simulink model "case5"  (R2024b)
settings: Solver=FixedStepAuto  StartTime=0  StopTime=1  FixedStep=1e-7  RelTol=1e-3
values from neighbouring files (symbols this model uses):
  SG_D_1_D = 0.01056    [IEEE9_case_parameters.m]    (also in case1_parameters.m; case2_parameters.m; case3_parameters.m; case4_parameters.m)
  SG_D_1_EnableSaturation = 0    [IEEE9_case_parameters.m]    (also in case1_parameters.m; case2_parameters.m; case3_parameters.m; case4_parameters.m)
  SG_D_1_f0 = 60    [IEEE9_case_parameters.m]    (also in case1_parameters.m; case2_parameters.m; case3_parameters.m; case4_parameters.m)
  SG_D_1_H = 7.5    [IEEE9_case_parameters.m]    (also in case1_parameters.m; case2_parameters.m; case3_parameters.m; case4_parameters.m)
  SG_D_1_K_A = 20    [IEEE9_case_parameters.m]    (also in case1_parameters.m; case2_parameters.m; case3_parameters.m; case4_parameters.m)
  SG_D_1_K_E = 1.000000e+1    (= 10)    [IEEE9_case_parameters.m]    (also in case1_parameters.m; case2_parameters.m; case3_parameters.m; case4_parameters.m)
  SG_D_1_K_F = 2.363    [IEEE9_case_parameters.m]    (also in case1_parameters.m; case2_parameters.m; case3_parameters.m; case4_parameters.m)
  SG_D_1_K_s = 0.5    [IEEE9_case_parameters.m]    (also in case1_parameters.m = 5; case2_parameters.m = 5; case3_parameters.m = 5; case4_parameters.m = 5)
  SG_D_1_R_a = 0.001088    [IEEE9_case_parameters.m]    (also in case1_parameters.m; case2_parameters.m; case3_parameters.m; case4_parameters.m)
  SG_D_1_S_A = 1    [IEEE9_case_parameters.m]    (also in case1_parameters.m; case2_parameters.m; case3_parameters.m; case4_parameters.m)
  SG_D_1_S_B = 0.103    [IEEE9_case_parameters.m]    (also in case1_parameters.m; case2_parameters.m; case3_parameters.m; case4_parameters.m)
  SG_D_1_S_N = 10.659857    [IEEE9_case_parameters.m]    (also in case1_parameters.m; case2_parameters.m; case3_parameters.m; case4_parameters.m)
  SG_D_1_SpeedPara = 200    [IEEE9_case_parameters.m]    (also in case1_parameters.m; case2_parameters.m; case3_parameters.m; case4_parameters.m)
  SG_D_1_T_0 = 0.720173    [IEEE9_case_parameters.m]    (also in case1_parameters.m = 0.755522; case2_parameters.m = 0.808931; case3_parameters.m = 0.869402; case4_parameters.m = 0.729316)
  SG_D_1_T_1 = 0.3    [IEEE9_case_parameters.m]    (also in case1_parameters.m; case2_parameters.m; case3_parameters.m; case4_parameters.m)
  SG_D_1_T_2 = 0.05    [IEEE9_case_parameters.m]    (also in case1_parameters.m; case2_parameters.m; case3_parameters.m; case4_parameters.m)
  SG_D_1_T_3 = 0.02    [IEEE9_case_parameters.m]    (also in case1_parameters.m; case2_parameters.m; case3_parameters.m; case4_parameters.m)
  SG_D_1_T_4 = 0.005    [IEEE9_case_parameters.m]    (also in case1_parameters.m; case2_parameters.m; case3_parameters.m; case4_parameters.m)
  SG_D_1_T_A = 0.02    [IEEE9_case_parameters.m]    (also in case1_parameters.m; case2_parameters.m; case3_parameters.m; case4_parameters.m)
  SG_D_1_T_dd = 8.000000e+0    (= 8)    [IEEE9_case_parameters.m]    (also in case1_parameters.m; case2_parameters.m; case3_parameters.m; case4_parameters.m)
  SG_D_1_T_ddd = 0.04    [IEEE9_case_parameters.m]    (also in case1_parameters.m; case2_parameters.m; case3_parameters.m; case4_parameters.m)
  SG_D_1_T_E = 0.314    [IEEE9_case_parameters.m]    (also in case1_parameters.m; case2_parameters.m; case3_parameters.m; case4_parameters.m)
  SG_D_1_T_F = 0.35    [IEEE9_case_parameters.m]    (also in case1_parameters.m; case2_parameters.m; case3_parameters.m; case4_parameters.m)
  SG_D_1_T_qd = 0.8    [IEEE9_case_parameters.m]    (also in case1_parameters.m; case2_parameters.m; case3_parameters.m; case4_parameters.m)
  SG_D_1_T_qdd = 0.02    [IEEE9_case_parameters.m]    (also in case1_parameters.m; case2_parameters.m; case3_parameters.m; case4_parameters.m)
  SG_D_1_T_speed = 0.1    [IEEE9_case_parameters.m]    (also in case1_parameters.m = 200; case2_parameters.m = 200; case3_parameters.m = 200; case4_parameters.m = 200)
  SG_D_1_T_w = 0.5    [IEEE9_case_parameters.m]    (also in case1_parameters.m; case2_parameters.m; case3_parameters.m; case4_parameters.m)
  SG_D_1_V_ref = 1.990276    [IEEE9_case_parameters.m]    (also in case1_parameters.m = 2.042296; case2_parameters.m = 2.051388; case3_parameters.m = 2.089584; case4_parameters.m = 2.01845)
  SG_D_1_w_ref = 376.991118    [IEEE9_case_parameters.m]    (also in case1_parameters.m; case2_parameters.m; case3_parameters.m; case4_parameters.m)
  SG_D_1_wb = 6.000000e+1    (= 60)    [IEEE9_case_parameters.m]    (also in case1_parameters.m; case2_parameters.m; case3_parameters.m; case4_parameters.m)
  SG_D_1_x_d = 1.9    [IEEE9_case_parameters.m]    (also in case1_parameters.m; case2_parameters.m; case3_parameters.m; case4_parameters.m)
  SG_D_1_x_dd = 0.302    [IEEE9_case_parameters.m]    (also in case1_parameters.m; case2_parameters.m; case3_parameters.m; case4_parameters.m)
  SG_D_1_x_ddd = 0.204    [IEEE9_case_parameters.m]    (also in case1_parameters.m; case2_parameters.m; case3_parameters.m; case4_parameters.m)
  SG_D_1_x_l = 0.05    [IEEE9_case_parameters.m]    (also in case1_parameters.m; case2_parameters.m; case3_parameters.m; case4_parameters.m)
  SG_D_1_x_q = 1.3    [IEEE9_case_parameters.m]    (also in case1_parameters.m; case2_parameters.m; case3_parameters.m; case4_parameters.m)
  SG_D_1_x_qd = 0.5    [IEEE9_case_parameters.m]    (also in case1_parameters.m; case2_parameters.m; case3_parameters.m; case4_parameters.m)
  SG_D_1_x_qdd = 0.3    [IEEE9_case_parameters.m]    (also in case1_parameters.m; case2_parameters.m; case3_parameters.m; case4_parameters.m)
  SG_D_2_D = 0.02    [IEEE9_case_parameters.m]    (also in case1_parameters.m; case2_parameters.m; case3_parameters.m; case4_parameters.m)
  SG_D_2_EnableSaturation = 0    [IEEE9_case_parameters.m]    (also in case1_parameters.m; case2_parameters.m; case3_parameters.m; case4_parameters.m)
  SG_D_2_f0 = 60    [IEEE9_case_parameters.m]    (also in case1_parameters.m; case2_parameters.m; case3_parameters.m; case4_parameters.m)
  SG_D_2_H = 8.000000e+0    (= 8)    [IEEE9_case_parameters.m]    (also in case1_parameters.m; case2_parameters.m; case3_parameters.m; case4_parameters.m)
  SG_D_2_K_A = 20    [IEEE9_case_parameters.m]    (also in case1_parameters.m; case2_parameters.m; case3_parameters.m; case4_parameters.m)
  SG_D_2_K_E = 1.000000e+1    (= 10)    [IEEE9_case_parameters.m]    (also in case1_parameters.m; case2_parameters.m; case3_parameters.m; case4_parameters.m)
  SG_D_2_K_F = 2.363    [IEEE9_case_parameters.m]    (also in case1_parameters.m; case2_parameters.m; case3_parameters.m; case4_parameters.m)
  SG_D_2_K_s = 0.5    [IEEE9_case_parameters.m]    (also in case1_parameters.m = 4; case2_parameters.m = 4; case3_parameters.m = 4; case4_parameters.m = 4)
  SG_D_2_R_a = 0.001088    [IEEE9_case_parameters.m]    (also in case1_parameters.m; case2_parameters.m; case3_parameters.m; case4_parameters.m)
  SG_D_2_S_A = 1    [IEEE9_case_parameters.m]    (also in case1_parameters.m; case2_parameters.m; case3_parameters.m; case4_parameters.m)
  SG_D_2_S_B = 0.103    [IEEE9_case_parameters.m]    (also in case1_parameters.m; case2_parameters.m; case3_parameters.m; case4_parameters.m)
  SG_D_2_S_N = 10.659857    [IEEE9_case_parameters.m]    (also in case1_parameters.m; case2_parameters.m; case3_parameters.m; case4_parameters.m)
  SG_D_2_SpeedPara = 200    [IEEE9_case_parameters.m]    (also in case1_parameters.m; case2_parameters.m; case3_parameters.m; case4_parameters.m)
  SG_D_2_T_0 = 1.632913    [IEEE9_case_parameters.m]    (also in case1_parameters.m = 1.632925; case2_parameters.m = 1.632915; case3_parameters.m = 1.632914; case4_parameters.m = 1.632927)
  SG_D_2_T_1 = 0.2    [IEEE9_case_parameters.m]    (also in case1_parameters.m; case2_parameters.m; case3_parameters.m; case4_parameters.m)
  SG_D_2_T_2 = 0.05    [IEEE9_case_parameters.m]    (also in case1_parameters.m; case2_parameters.m; case3_parameters.m; case4_parameters.m)
  SG_D_2_T_3 = 0.02    [IEEE9_case_parameters.m]    (also in case1_parameters.m; case2_parameters.m; case3_parameters.m; case4_parameters.m)
  SG_D_2_T_4 = 0.005    [IEEE9_case_parameters.m]    (also in case1_parameters.m; case2_parameters.m; case3_parameters.m; case4_parameters.m)
  SG_D_2_T_A = 0.02    [IEEE9_case_parameters.m]    (also in case1_parameters.m; case2_parameters.m; case3_parameters.m; case4_parameters.m)
  SG_D_2_T_dd = 7.9    [IEEE9_case_parameters.m]    (also in case1_parameters.m; case2_parameters.m; case3_parameters.m; case4_parameters.m)
  SG_D_2_T_ddd = 0.04    [IEEE9_case_parameters.m]    (also in case1_parameters.m; case2_parameters.m; case3_parameters.m; case4_parameters.m)
  SG_D_2_T_E = 0.314    [IEEE9_case_parameters.m]    (also in case1_parameters.m; case2_parameters.m; case3_parameters.m; case4_parameters.m)
  SG_D_2_T_F = 0.35    [IEEE9_case_parameters.m]    (also in case1_parameters.m; case2_parameters.m; case3_parameters.m; case4_parameters.m)
  SG_D_2_T_qd = 0.8    [IEEE9_case_parameters.m]    (also in case1_parameters.m; case2_parameters.m; case3_parameters.m; case4_parameters.m)
  SG_D_2_T_qdd = 0.015    [IEEE9_case_parameters.m]    (also in case1_parameters.m; case2_parameters.m; case3_parameters.m; case4_parameters.m)
  SG_D_2_T_speed = 0.1    [IEEE9_case_parameters.m]    (also in case1_parameters.m = 150; case2_parameters.m = 150; case3_parameters.m = 150; case4_parameters.m = 150)
  SG_D_2_T_w = 0.35    [IEEE9_case_parameters.m]    (also in case1_parameters.m; case2_parameters.m; case3_parameters.m; case4_parameters.m)
  SG_D_2_V_ref = 2.58547    [IEEE9_case_parameters.m]    (also in case1_parameters.m = 2.597896; case2_parameters.m = 2.587136; case3_parameters.m = 2.586042; case4_parameters.m = 2.599679)
  SG_D_2_w_ref = 376.991118    [IEEE9_case_parameters.m]    (also in case1_parameters.m; case2_parameters.m; case3_parameters.m; case4_parameters.m)
  SG_D_2_wb = 6.000000e+1    (= 60)    [IEEE9_case_parameters.m]    (also in case1_parameters.m; case2_parameters.m; case3_parameters.m; case4_parameters.m)
  SG_D_2_x_d = 1.8    [IEEE9_case_parameters.m]    (also in case1_parameters.m; case2_parameters.m; case3_parameters.m; case4_parameters.m)
  SG_D_2_x_dd = 0.302    [IEEE9_case_parameters.m]    (also in case1_parameters.m; case2_parameters.m; case3_parameters.m; case4_parameters.m)
  SG_D_2_x_ddd = 0.204    [IEEE9_case_parameters.m]    (also in case1_parameters.m; case2_parameters.m; case3_parameters.m; case4_parameters.m)
  SG_D_2_x_l = 0.05    [IEEE9_case_parameters.m]    (also in case1_parameters.m; case2_parameters.m; case3_parameters.m; case4_parameters.m)
  SG_D_2_x_q = 1.25    [IEEE9_case_parameters.m]    (also in case1_parameters.m; case2_parameters.m; case3_parameters.m; case4_parameters.m)
  SG_D_2_x_qd = 0.5    [IEEE9_case_parameters.m]    (also in case1_parameters.m; case2_parameters.m; case3_parameters.m; case4_parameters.m)
  SG_D_2_x_qdd = 0.3    [IEEE9_case_parameters.m]    (also in case1_parameters.m; case2_parameters.m; case3_parameters.m; case4_parameters.m)
  SG_D_3_D = 0.02    [IEEE9_case_parameters.m]    (also in case1_parameters.m; case2_parameters.m; case3_parameters.m; case4_parameters.m)
  SG_D_3_EnableSaturation = 0    [IEEE9_case_parameters.m]    (also in case1_parameters.m; case2_parameters.m; case3_parameters.m; case4_parameters.m)
  SG_D_3_f0 = 60    [IEEE9_case_parameters.m]    (also in case1_parameters.m; case2_parameters.m; case3_parameters.m; case4_parameters.m)
  SG_D_3_H = 7.7    [IEEE9_case_parameters.m]    (also in case1_parameters.m; case2_parameters.m; case3_parameters.m; case4_parameters.m)
  SG_D_3_K_A = 20    [IEEE9_case_parameters.m]    (also in case1_parameters.m; case2_parameters.m; case3_parameters.m; case4_parameters.m)
  SG_D_3_K_E = 1.000000e+1    (= 10)    [IEEE9_case_parameters.m]    (also in case1_parameters.m; case2_parameters.m; case3_parameters.m; case4_parameters.m)
  SG_D_3_K_F = 2.363    [IEEE9_case_parameters.m]    (also in case1_parameters.m; case2_parameters.m; case3_parameters.m; case4_parameters.m)
  SG_D_3_K_s = 0.2    [IEEE9_case_parameters.m]    (also in case1_parameters.m = 2; case2_parameters.m = 2; case3_parameters.m = 2; case4_parameters.m = 2)
  SG_D_3_R_a = 0.001088    [IEEE9_case_parameters.m]    (also in case1_parameters.m; case2_parameters.m; case3_parameters.m; case4_parameters.m)
  SG_D_3_S_A = 1    [IEEE9_case_parameters.m]    (also in case1_parameters.m; case2_parameters.m; case3_parameters.m; case4_parameters.m)
  SG_D_3_S_B = 0.103    [IEEE9_case_parameters.m]    (also in case1_parameters.m; case2_parameters.m; case3_parameters.m; case4_parameters.m)
  SG_D_3_S_N = 10.659857    [IEEE9_case_parameters.m]    (also in case1_parameters.m; case2_parameters.m; case3_parameters.m; case4_parameters.m)
  SG_D_3_SpeedPara = 200    [IEEE9_case_parameters.m]    (also in case1_parameters.m; case2_parameters.m; case3_parameters.m; case4_parameters.m)
  SG_D_3_T_0 = 0.850788    [IEEE9_case_parameters.m]    (also in case1_parameters.m = 0.850786; case2_parameters.m = 0.850787; case3_parameters.m; case4_parameters.m = 0.850786)
  SG_D_3_T_1 = 0.2    [IEEE9_case_parameters.m]    (also in case1_parameters.m; case2_parameters.m; case3_parameters.m; case4_parameters.m)
  SG_D_3_T_2 = 0.05    [IEEE9_case_parameters.m]    (also in case1_parameters.m; case2_parameters.m; case3_parameters.m; case4_parameters.m)
  SG_D_3_T_3 = 0.02    [IEEE9_case_parameters.m]    (also in case1_parameters.m; case2_parameters.m; case3_parameters.m; case4_parameters.m)
  SG_D_3_T_4 = 0.005    [IEEE9_case_parameters.m]    (also in case1_parameters.m; case2_parameters.m; case3_parameters.m; case4_parameters.m)
  SG_D_3_T_A = 0.02    [IEEE9_case_parameters.m]    (also in case1_parameters.m; case2_parameters.m; case3_parameters.m; case4_parameters.m)
  SG_D_3_T_dd = 8.1    [IEEE9_case_parameters.m]    (also in case1_parameters.m; case2_parameters.m; case3_parameters.m; case4_parameters.m)
  SG_D_3_T_ddd = 0.04    [IEEE9_case_parameters.m]    (also in case1_parameters.m; case2_parameters.m; case3_parameters.m; case4_parameters.m)
  SG_D_3_T_E = 0.314    [IEEE9_case_parameters.m]    (also in case1_parameters.m; case2_parameters.m; case3_parameters.m; case4_parameters.m)
  SG_D_3_T_F = 0.35    [IEEE9_case_parameters.m]    (also in case1_parameters.m; case2_parameters.m; case3_parameters.m; case4_parameters.m)
  SG_D_3_T_qd = 0.8    [IEEE9_case_parameters.m]    (also in case1_parameters.m; case2_parameters.m; case3_parameters.m; case4_parameters.m)
  SG_D_3_T_qdd = 0.015    [IEEE9_case_parameters.m]    (also in case1_parameters.m; case2_parameters.m; case3_parameters.m; case4_parameters.m)
  SG_D_3_T_speed = 0.1    [IEEE9_case_parameters.m]    (also in case1_parameters.m = 180; case2_parameters.m = 180; case3_parameters.m = 180; case4_parameters.m = 180)
  SG_D_3_T_w = 0.4    [IEEE9_case_parameters.m]    (also in case1_parameters.m; case2_parameters.m; case3_parameters.m; case4_parameters.m)
  SG_D_3_V_ref = 1.892727    [IEEE9_case_parameters.m]    (also in case1_parameters.m = 1.906439; case2_parameters.m = 1.895535; case3_parameters.m = 1.892105; case4_parameters.m = 1.906598)
  SG_D_3_w_ref = 376.991118    [IEEE9_case_parameters.m]    (also in case1_parameters.m; case2_parameters.m; case3_parameters.m; case4_parameters.m)
  SG_D_3_wb = 6.000000e+1    (= 60)    [IEEE9_case_parameters.m]    (also in case1_parameters.m; case2_parameters.m; case3_parameters.m; case4_parameters.m)
  SG_D_3_x_d = 1.85    [IEEE9_case_parameters.m]    (also in case1_parameters.m; case2_parameters.m; case3_parameters.m; case4_parameters.m)
  SG_D_3_x_dd = 0.302    [IEEE9_case_parameters.m]    (also in case1_parameters.m; case2_parameters.m; case3_parameters.m; case4_parameters.m)
  SG_D_3_x_ddd = 0.204    [IEEE9_case_parameters.m]    (also in case1_parameters.m; case2_parameters.m; case3_parameters.m; case4_parameters.m)
  SG_D_3_x_l = 0.05    [IEEE9_case_parameters.m]    (also in case1_parameters.m; case2_parameters.m; case3_parameters.m; case4_parameters.m)
  SG_D_3_x_q = 1.2    [IEEE9_case_parameters.m]    (also in case1_parameters.m; case2_parameters.m; case3_parameters.m; case4_parameters.m)
  SG_D_3_x_qd = 0.5    [IEEE9_case_parameters.m]    (also in case1_parameters.m; case2_parameters.m; case3_parameters.m; case4_parameters.m)
  SG_D_3_x_qdd = 0.3    [IEEE9_case_parameters.m]    (also in case1_parameters.m; case2_parameters.m; case3_parameters.m; case4_parameters.m)
(part 7 of 12)

== system case5/SG_D_2/T_e_SG_D_2_block ==
  note: T_e_SG_D_2 in case5
      | $-\frac{\psi _{d,\mathrm{SG},D,2}\,\left(\psi _{q,\mathrm{SG},D,2}+\frac{\psi _{\mathrm{gq},\mathrm{SG},D,2}\,\left(x_{l}-x_{\mathrm{qdd}}\right)}{x_{l}-x_{\mathrm{qd}}}+\frac{\psi _{\mathrm{kq},\mathrm{SG},D,2}\,\left(x_{\mathrm{qd}}-x_{\mathrm{qdd}}\right)}{x_{l}-x_{\mathrm{qd}}}\right)}{x_{\mathrm{qdd}}}-\frac{\psi _{q,\mathrm{SG},D,2}\,\left(\frac{\psi _{\mathrm{1d},\mathrm{SG},D,2}\,\left(x_{\mathrm{dd}}-x_{\mathrm{ddd}}\right)}{x_{\mathrm{dd}}-x_{l}}-\psi _{d,\mathrm{SG},D,2}+\frac{\psi _{\mathrm{fd},\mathrm{SG},D,2}\,\left(x_{\mathrm{ddd}}-x_{l}\right)}{x_{\mathrm{dd}}-x_{l}}\right)}{x_{\mathrm{ddd}}}$
      | Automatically generated on 2025-10-31 19:11:59 .
  State_psi_d_SG_D_2_8764f : Inport
  State_psi_gq_SG_D_2_1f7cf : Inport  Port=2
  State_psi_kq_SG_D_2_b1f64 : Inport  Port=3
  State_psi_q_SG_D_2_7d7d0 : Inport  Port=4
  State_psi_q_SG_D_2_860cc : Inport  Port=5
  State_psi_1d_SG_D_2_4989b : Inport  Port=6
  State_psi_d_SG_D_2_cc96c : Inport  Port=7
  State_psi_fd_SG_D_2_f288a : Inport  Port=8
  Add_4ea1b : Sum
  Add_6a2e1 : Sum
  Add_77a1d : Sum
  Add_7defb : Sum
  Add_a1766 : Sum
  Add_fd560 : Sum
  Constant_-1_6d645 : Constant  Value=-1
  Constant_-1_6fd96 : Constant  Value=-1
  Constant_-1_a2653 : Constant  Value=-1
  Constant_-1_bed53 : Constant  Value=-1
  Constant_-1_c9aec : Constant  Value=-1
  Constant_x_dd_110ca : Constant  Value=x_dd
  Constant_x_dd_1b426 : Constant  Value=x_dd
  Constant_x_dd_603c3 : Constant  Value=x_dd
  Constant_x_ddd_039fd : Constant  Value=x_ddd
  Constant_x_ddd_2ebf2 : Constant  Value=x_ddd
  Constant_x_ddd_fde4e : Constant  Value=x_ddd
  Constant_x_l_026ea : Constant  Value=x_l
  Constant_x_l_085f5 : Constant  Value=x_l
  Constant_x_l_13a0c : Constant  Value=x_l
  Constant_x_l_3979a : Constant  Value=x_l
  Constant_x_l_ba3c7 : Constant  Value=x_l
  Constant_x_l_ec106 : Constant  Value=x_l
  Constant_x_qd_460b0 : Constant  Value=x_qd
  Constant_x_qd_54b57 : Constant  Value=x_qd
  Constant_x_qd_ab5a4 : Constant  Value=x_qd
  Constant_x_qdd_30d29 : Constant  Value=x_qdd
  Constant_x_qdd_b0a37 : Constant  Value=x_qdd
  Constant_x_qdd_b570c : Constant  Value=x_qdd
  Divide_13c40 : Product  Inputs=*/
  Divide_4a1e5 : Product  Inputs=*/
  Divide_838a3 : Product  Inputs=*/
  Divide_9315b : Product  Inputs=*/
  Divide_db35b : Product  Inputs=*/
  Divide_fdf5d : Product  Inputs=*/
  Product_176e1 : Product
  Product_33191 : Product
  Product_43418 : Product
  Product_7e007 : Product
  Product_84689 : Product
  Product_85a87 : Product
  Product_8d2ff : Product
  Product_a5a2e : Product
  Product_ac49e : Product
  Product_b4402 : Product
  Product_dabe4 : Product
  Subtract_0e07a : Sum  Inputs=+-
  Subtract_45d12 : Sum  Inputs=+-
  Subtract_70a71 : Sum  Inputs=+-
  Subtract_7eb8f : Sum  Inputs=+-
  Subtract_970c6 : Sum  Inputs=+-
  Subtract_e5e99 : Sum  Inputs=+-
  Subtract_ef4a2 : Sum  Inputs=+-
  Blockout_T_e_SG_D_2_32ea4 : Outport
  wires:
  Constant_-1_6fd96/1 -> Product_7e007/1
  Divide_fdf5d/1 -> Subtract_e5e99/1
  Constant_-1_bed53/1 -> Product_176e1/1
  Constant_x_l_085f5/1 -> Product_176e1/2
  Constant_x_qd_460b0/1 -> Subtract_45d12/1
  Product_33191/1 -> Divide_fdf5d/1
  Product_176e1/1 -> Add_6a2e1/1
  Divide_13c40/1 -> Subtract_970c6/2
  Constant_x_qdd_b0a37/1 -> Subtract_45d12/2
  Constant_x_qdd_30d29/1 -> Divide_4a1e5/2
  Constant_x_ddd_2ebf2/1 -> Subtract_7eb8f/2
  Constant_x_qdd_b570c/1 -> Add_6a2e1/2
  Constant_x_l_ba3c7/1 -> Product_7e007/2
  Constant_-1_c9aec/1 -> Product_84689/1
  Constant_x_l_3979a/1 -> Product_84689/2
  Constant_-1_a2653/1 -> Product_8d2ff/1
  State_psi_1d_SG_D_2_4989b/1 -> Product_8d2ff/2
  Constant_x_dd_603c3/1 -> Subtract_7eb8f/1
  Divide_db35b/1 -> Subtract_e5e99/2
  State_psi_gq_SG_D_2_1f7cf/1 -> Product_33191/1
  Add_6a2e1/1 -> Product_33191/2
  Subtract_e5e99/1 -> Add_a1766/1
  Constant_x_dd_1b426/1 -> Subtract_ef4a2/1
  Product_7e007/1 -> Add_4ea1b/1
  Product_43418/1 -> Product_b4402/1
  Constant_x_qd_ab5a4/1 -> Add_4ea1b/2
  State_psi_kq_SG_D_2_b1f64/1 -> Product_dabe4/1
  Subtract_45d12/1 -> Product_dabe4/2
  Product_84689/1 -> Add_77a1d/1
  State_psi_q_SG_D_2_860cc/1 -> Product_ac49e/1
  Constant_x_qd_54b57/1 -> Add_77a1d/2
  Product_8d2ff/1 -> Product_85a87/1
  Divide_9315b/1 -> Add_7defb/2
  Subtract_7eb8f/1 -> Product_85a87/2
  Constant_x_l_13a0c/1 -> Subtract_ef4a2/2
  Constant_x_ddd_039fd/1 -> Subtract_70a71/1
  Constant_x_dd_110ca/1 -> Subtract_0e07a/1
  Constant_x_l_ec106/1 -> Subtract_70a71/2
  Add_7defb/1 -> Blockout_T_e_SG_D_2_32ea4/1
  Add_4ea1b/1 -> Divide_fdf5d/2
  Product_dabe4/1 -> Divide_db35b/1
  Product_b4402/1 -> Divide_4a1e5/1
  State_psi_d_SG_D_2_8764f/1 -> Product_43418/2
  Add_77a1d/1 -> Divide_db35b/2
  Product_85a87/1 -> Divide_838a3/1
  Subtract_ef4a2/1 -> Divide_838a3/2
  Constant_x_l_026ea/1 -> Subtract_0e07a/2
  State_psi_fd_SG_D_2_f288a/1 -> Product_a5a2e/1
  Constant_x_ddd_fde4e/1 -> Divide_9315b/2
  Product_ac49e/1 -> Divide_9315b/1
  Subtract_70a71/1 -> Product_a5a2e/2
  Divide_838a3/1 -> Add_fd560/1
  State_psi_d_SG_D_2_cc96c/1 -> Add_fd560/2
  Add_fd560/1 -> Subtract_970c6/1
  Product_a5a2e/1 -> Divide_13c40/1
  Subtract_0e07a/1 -> Divide_13c40/2
  Constant_-1_6d645/1 -> Product_43418/1
  State_psi_q_SG_D_2_7d7d0/1 -> Add_a1766/2
  Add_a1766/1 -> Product_b4402/2
  Subtract_970c6/1 -> Product_ac49e/2
  Divide_4a1e5/1 -> Add_7defb/1

== system case5/SG_D_2/d_E_fd_SG_D_2_block ==
  note: d_E_fd_SG_D_2 in case5
      | $\frac{V_{f,\mathrm{SG},D,2}-E_{\mathrm{fd},\mathrm{SG},D,2}\,K_{E}}{T_{E}}$
      | Automatically generated on 2025-10-31 19:11:39 .
  State_E_fd_SG_D_2_808fd : Inport
  State_V_f_SG_D_2_4e077 : Inport  Port=2
  Add_b92ab : Sum
  Constant_-1_6f407 : Constant  Value=-1
  Constant_K_E_a9583 : Constant  Value=K_E
  Constant_T_E_299c6 : Constant  Value=T_E
  Divide_a8a3d : Product  Inputs=*/
  Product_10ad6 : Product
  Product_f58d4 : Product
  Blockout_d_E_fd_SG_D_2_55c73 : Outport
  wires:
  Constant_-1_6f407/1 -> Product_f58d4/1
  State_E_fd_SG_D_2_808fd/1 -> Product_f58d4/2
  Product_f58d4/1 -> Product_10ad6/1
  Constant_K_E_a9583/1 -> Product_10ad6/2
  Product_10ad6/1 -> Add_b92ab/1
  Constant_T_E_299c6/1 -> Divide_a8a3d/2
  State_V_f_SG_D_2_4e077/1 -> Add_b92ab/2
  Add_b92ab/1 -> Divide_a8a3d/1
  Divide_a8a3d/1 -> Blockout_d_E_fd_SG_D_2_55c73/1

== system case5/SG_D_2/d_Px_1_SG_D_2_block ==
  note: d_Px_1_SG_D_2 in case5
      | $\frac{w_{\mathrm{SG},D,2}-2\,\pi \,f_{0}}{T_{w}}-\frac{\mathrm{Px}_{1,\mathrm{SG},D,2}}{T_{w}}$
      | Automatically generated on 2025-10-31 19:11:41 .
  State_Px_1_SG_D_2_dcfec : Inport
  State_w_SG_D_2_0a872 : Inport  Port=2
  Add_7fc50 : Sum
  Add_fd0af : Sum
  Constant_-1_18e10 : Constant  Value=-1
  Constant_-2.0_af387 : Constant  Value=-2.0
  Constant_T_w_4ffa8 : Constant  Value=T_w
  Constant_T_w_f48b1 : Constant  Value=T_w
  Constant_f0_97983 : Constant  Value=f0
  Constant_pi_be5bb : Constant  Value=pi
  Divide_2a4bc : Product  Inputs=*/
  Divide_789a1 : Product  Inputs=*/
  Product_0c877 : Product
  Product_1a8c9 : Product
  Product_e895c : Product
  Blockout_d_Px_1_SG_D_2_3a836 : Outport
  wires:
  Constant_-2.0_af387/1 -> Product_1a8c9/1
  State_w_SG_D_2_0a872/1 -> Add_fd0af/2
  Constant_pi_be5bb/1 -> Product_1a8c9/2
  Product_1a8c9/1 -> Product_e895c/1
  Constant_f0_97983/1 -> Product_e895c/2
  Constant_-1_18e10/1 -> Product_0c877/1
  State_Px_1_SG_D_2_dcfec/1 -> Product_0c877/2
  Product_e895c/1 -> Add_fd0af/1
  Product_0c877/1 -> Divide_2a4bc/1
  Constant_T_w_4ffa8/1 -> Divide_2a4bc/2
  Add_fd0af/1 -> Divide_789a1/1
  Constant_T_w_f48b1/1 -> Divide_789a1/2
  Divide_2a4bc/1 -> Add_7fc50/1
  Divide_789a1/1 -> Add_7fc50/2
  Add_7fc50/1 -> Blockout_d_Px_1_SG_D_2_3a836/1

== system case5/SG_D_2/d_Px_2_SG_D_2_block ==
  note: d_Px_2_SG_D_2 in case5
      | $\frac{\mathrm{Px}_{1,\mathrm{SG},D,2}-T_{2}\,\left(\frac{\mathrm{Px}_{1,\mathrm{SG},D,2}}{T_{w}}-\frac{w_{\mathrm{SG},D,2}-2\,\pi \,f_{0}}{T_{w}}\right)}{T_{1}}-\frac{\mathrm{Px}_{2,\mathrm{SG},D,2}}{T_{1}}$
      | Automatically generated on 2025-10-31 19:11:43 .
  State_Px_2_SG_D_2_3d84e : Inport
  State_Px_1_SG_D_2_e7928 : Inport  Port=2
  State_Px_1_SG_D_2_6b838 : Inport  Port=3
  State_w_SG_D_2_c4bce : Inport  Port=4
  Add_00813 : Sum
  Add_8757f : Sum
  Add_8a97d : Sum
  Add_952a4 : Sum
  Constant_-1_2daee : Constant  Value=-1
  Constant_-1_d1ca8 : Constant  Value=-1
  Constant_-2.0_4ab62 : Constant  Value=-2.0
  Constant_T_1_280f9 : Constant  Value=T_1
  Constant_T_1_6f68d : Constant  Value=T_1
  Constant_T_2_6ecb6 : Constant  Value=T_2
  Constant_T_w_041db : Constant  Value=T_w
  Constant_T_w_4627f : Constant  Value=T_w
  Constant_f0_1ecde : Constant  Value=f0
  Constant_pi_53a50 : Constant  Value=pi
  Divide_01d62 : Product  Inputs=*/
  Divide_210ef : Product  Inputs=*/
  Divide_4f18f : Product  Inputs=*/
  Divide_ac4e2 : Product  Inputs=*/
  Product_3c12f : Product
  Product_6f61c : Product
  Product_9cbe4 : Product
  Product_a935b : Product
  Product_be960 : Product
  Blockout_d_Px_2_SG_D_2_04e36 : Outport
  wires:
  Constant_-1_d1ca8/1 -> Product_9cbe4/1
  Constant_-2.0_4ab62/1 -> Product_3c12f/1
  Product_be960/1 -> Add_952a4/2
  State_w_SG_D_2_c4bce/1 -> Add_8a97d/2
  Constant_pi_53a50/1 -> Product_3c12f/2
  Product_3c12f/1 -> Product_a935b/1
  State_Px_1_SG_D_2_6b838/1 -> Product_6f61c/2
  Constant_f0_1ecde/1 -> Product_a935b/2
  State_Px_2_SG_D_2_3d84e/1 -> Product_9cbe4/2
  Constant_-1_2daee/1 -> Product_6f61c/1
  Product_a935b/1 -> Add_8a97d/1
  Product_6f61c/1 -> Divide_210ef/1
  Constant_T_w_041db/1 -> Divide_210ef/2
  Add_8a97d/1 -> Divide_4f18f/1
  Constant_T_w_4627f/1 -> Divide_4f18f/2
  Divide_210ef/1 -> Add_8757f/1
  Divide_4f18f/1 -> Add_8757f/2
  Constant_T_2_6ecb6/1 -> Product_be960/1
  Add_8757f/1 -> Product_be960/2
  State_Px_1_SG_D_2_e7928/1 -> Add_952a4/1
  Product_9cbe4/1 -> Divide_ac4e2/1
  Constant_T_1_280f9/1 -> Divide_ac4e2/2
  Add_952a4/1 -> Divide_01d62/1
  Constant_T_1_6f68d/1 -> Divide_01d62/2
  Divide_ac4e2/1 -> Add_00813/1
  Divide_01d62/1 -> Add_00813/2
  Add_00813/1 -> Blockout_d_Px_2_SG_D_2_04e36/1

== system case5/SG_D_2/d_Px_3_SG_D_2_block ==
  note: d_Px_3_SG_D_2 in case5
      | $\frac{\mathrm{Px}_{2,\mathrm{SG},D,2}+T_{4}\,\left(\frac{\mathrm{Px}_{1,\mathrm{SG},D,2}-T_{2}\,\left(\frac{\mathrm{Px}_{1,\mathrm{SG},D,2}}{T_{w}}-\frac{w_{\mathrm{SG},D,2}-2\,\pi \,f_{0}}{T_{w}}\right)}{T_{1}}-\frac{\mathrm{Px}_{2,\mathrm{SG},D,2}}{T_{1}}\right)}{T_{3}}-\frac{\mathrm{Px}_{3,\mathrm{SG},D,2}}{T_{3}}$
      | Automatically generated on 2025-10-31 19:11:45 .
  State_Px_3_SG_D_2_615b8 : Inport
  State_Px_2_SG_D_2_ea741 : Inport  Port=2
  State_Px_2_SG_D_2_55edc : Inport  Port=3
  State_Px_1_SG_D_2_820be : Inport  Port=4
  State_Px_1_SG_D_2_81adf : Inport  Port=5
  State_w_SG_D_2_e9070 : Inport  Port=6
  Add_0c02d : Sum
  Add_3158f : Sum
  Add_4fdfa : Sum
  Add_6455c : Sum
  Add_eabaa : Sum
  Add_f9b5f : Sum
  Constant_-1_9126a : Constant  Value=-1
  Constant_-1_9489f : Constant  Value=-1
  Constant_-1_ca78e : Constant  Value=-1
  Constant_-2.0_ac31e : Constant  Value=-2.0
  Constant_T_1_10029 : Constant  Value=T_1
  Constant_T_1_13c66 : Constant  Value=T_1
  Constant_T_2_c8116 : Constant  Value=T_2
  Constant_T_3_c6817 : Constant  Value=T_3
  Constant_T_3_d860c : Constant  Value=T_3
  Constant_T_4_9c252 : Constant  Value=T_4
  Constant_T_w_8815c : Constant  Value=T_w
  Constant_T_w_ab9ec : Constant  Value=T_w
  Constant_f0_cbd55 : Constant  Value=f0
  Constant_pi_70a46 : Constant  Value=pi
  Divide_1514f : Product  Inputs=*/
  Divide_1df3f : Product  Inputs=*/
  Divide_2f4db : Product  Inputs=*/
  Divide_36895 : Product  Inputs=*/
  Divide_9d579 : Product  Inputs=*/
  Divide_addd2 : Product  Inputs=*/
  Product_8d7a1 : Product
  Product_b1d42 : Product
  Product_b6660 : Product
  Product_ba740 : Product
  Product_d1cf8 : Product
  Product_ee23a : Product
  Product_fb85f : Product
  Blockout_d_Px_3_SG_D_2_0e921 : Outport
  wires:
  Constant_-2.0_ac31e/1 -> Product_8d7a1/1
  State_w_SG_D_2_e9070/1 -> Add_4fdfa/2
  Add_eabaa/1 -> Divide_2f4db/1
  Constant_pi_70a46/1 -> Product_8d7a1/2
  Constant_-1_9489f/1 -> Product_fb85f/1
  Product_8d7a1/1 -> Product_b1d42/1
  State_Px_2_SG_D_2_55edc/1 -> Product_fb85f/2
  State_Px_1_SG_D_2_81adf/1 -> Product_d1cf8/2
  Divide_2f4db/1 -> Add_f9b5f/2
  Constant_f0_cbd55/1 -> Product_b1d42/2
  Constant_-1_9126a/1 -> Product_d1cf8/1
  Product_b1d42/1 -> Add_4fdfa/1
  Product_d1cf8/1 -> Divide_1df3f/1
  Constant_T_w_8815c/1 -> Divide_1df3f/2
  Divide_1514f/1 -> Add_f9b5f/1
  Add_4fdfa/1 -> Divide_36895/1
  Product_b6660/1 -> Add_0c02d/2
  Constant_T_w_ab9ec/1 -> Divide_36895/2
  Divide_1df3f/1 -> Add_6455c/1
  State_Px_1_SG_D_2_820be/1 -> Add_0c02d/1
  Divide_36895/1 -> Add_6455c/2
  Constant_-1_ca78e/1 -> Product_ee23a/1
  Constant_T_2_c8116/1 -> Product_b6660/1
  Add_6455c/1 -> Product_b6660/2
  Product_fb85f/1 -> Divide_9d579/1
  Constant_T_1_13c66/1 -> Divide_9d579/2
  Add_0c02d/1 -> Divide_addd2/1
  Constant_T_1_10029/1 -> Divide_addd2/2
  Divide_9d579/1 -> Add_3158f/1
  Divide_addd2/1 -> Add_3158f/2
  Constant_T_4_9c252/1 -> Product_ba740/1
  Add_3158f/1 -> Product_ba740/2
  State_Px_3_SG_D_2_615b8/1 -> Product_ee23a/2
  State_Px_2_SG_D_2_ea741/1 -> Add_eabaa/1
  Product_ba740/1 -> Add_eabaa/2
  Product_ee23a/1 -> Divide_1514f/1
  Constant_T_3_c6817/1 -> Divide_1514f/2
  Constant_T_3_d860c/1 -> Divide_2f4db/2
  Add_f9b5f/1 -> Blockout_d_Px_3_SG_D_2_0e921/1

== system case5/SG_D_2/d_R_f_SG_D_2_block ==
  note: d_R_f_SG_D_2 in case5
      | $-\frac{R_{f,\mathrm{SG},D,2}-\frac{E_{\mathrm{fd},\mathrm{SG},D,2}\,K_{F}}{T_{F}}}{T_{F}}$
      | Automatically generated on 2025-10-31 19:11:38 .
  State_E_fd_SG_D_2_65d60 : Inport
  State_R_f_SG_D_2_625bf : Inport  Port=2
  Constant_K_F_8c078 : Constant  Value=K_F
  Constant_T_F_a58c1 : Constant  Value=T_F
  Constant_T_F_f09bb : Constant  Value=T_F
  Divide_3b7b4 : Product  Inputs=*/
  Divide_81cba : Product  Inputs=*/
  Product_37f63 : Product
  Subtract_38e20 : Sum  Inputs=+-
  Blockout_d_R_f_SG_D_2_818dd : Outport
  wires:
  Constant_T_F_f09bb/1 -> Divide_3b7b4/2
  State_E_fd_SG_D_2_65d60/1 -> Product_37f63/1
  Constant_K_F_8c078/1 -> Product_37f63/2
  State_R_f_SG_D_2_625bf/1 -> Subtract_38e20/2
  Product_37f63/1 -> Divide_3b7b4/1
  Divide_3b7b4/1 -> Subtract_38e20/1
  Constant_T_F_a58c1/1 -> Divide_81cba/2
  Subtract_38e20/1 -> Divide_81cba/1
  Divide_81cba/1 -> Blockout_d_R_f_SG_D_2_818dd/1

== system case5/SG_D_2/d_T_m_SG_D_2_block ==
  note: d_T_m_SG_D_2 in case5
      | $-\frac{T_{m,\mathrm{SG},D,2}-T_{0}+\frac{\mathrm{SpeedPara}\,\left(w_{\mathrm{SG},D,2}-w_{\mathrm{ref}}\right)}{2\,f_{0}\,\pi }}{T_{\mathrm{speed}}}$
      | Automatically generated on 2025-10-31 19:11:28 .
  State_w_SG_D_2_ee856 : Inport
  State_T_m_SG_D_2_0b68a : Inport  Port=2
  Add_4c623 : Sum
  Add_d7e7d : Sum
  Constant_-1_7beba : Constant  Value=-1
  Constant_2.0_8024e : Constant  Value=2.0
  Constant_SpeedPara_13d3b : Constant  Value=SpeedPara
  Constant_T_0_5f1eb : Constant  Value=T_0
  Constant_T_speed_bed5c : Constant  Value=T_speed
  Constant_f0_62c1f : Constant  Value=f0
  Constant_pi_14469 : Constant  Value=pi
  Constant_w_ref_ef544 : Constant  Value=w_ref
  Divide_f0042 : Product  Inputs=*/
  Divide_f2c70 : Product  Inputs=*/
  Product_093fa : Product
  Product_6154c : Product
  Product_c4892 : Product
  Product_c5360 : Product
  Subtract_f335a : Sum  Inputs=+-
  Blockout_d_T_m_SG_D_2_8be19 : Outport
  wires:
  Constant_pi_14469/1 -> Product_c4892/2
  Constant_-1_7beba/1 -> Product_c5360/1
  Constant_w_ref_ef544/1 -> Add_4c623/2
  State_w_SG_D_2_ee856/1 -> Product_c5360/2
  Product_c5360/1 -> Add_4c623/1
  Add_d7e7d/1 -> Subtract_f335a/1
  Add_4c623/1 -> Product_6154c/2
  Constant_2.0_8024e/1 -> Product_c4892/1
  Constant_SpeedPara_13d3b/1 -> Product_6154c/1
  Product_c4892/1 -> Product_093fa/1
  Constant_f0_62c1f/1 -> Product_093fa/2
  Product_6154c/1 -> Divide_f0042/1
  Product_093fa/1 -> Divide_f0042/2
  Divide_f0042/1 -> Add_d7e7d/1
  Constant_T_0_5f1eb/1 -> Add_d7e7d/2
  State_T_m_SG_D_2_0b68a/1 -> Subtract_f335a/2
  Subtract_f335a/1 -> Divide_f2c70/1
  Constant_T_speed_bed5c/1 -> Divide_f2c70/2
  Divide_f2c70/1 -> Blockout_d_T_m_SG_D_2_8be19/1

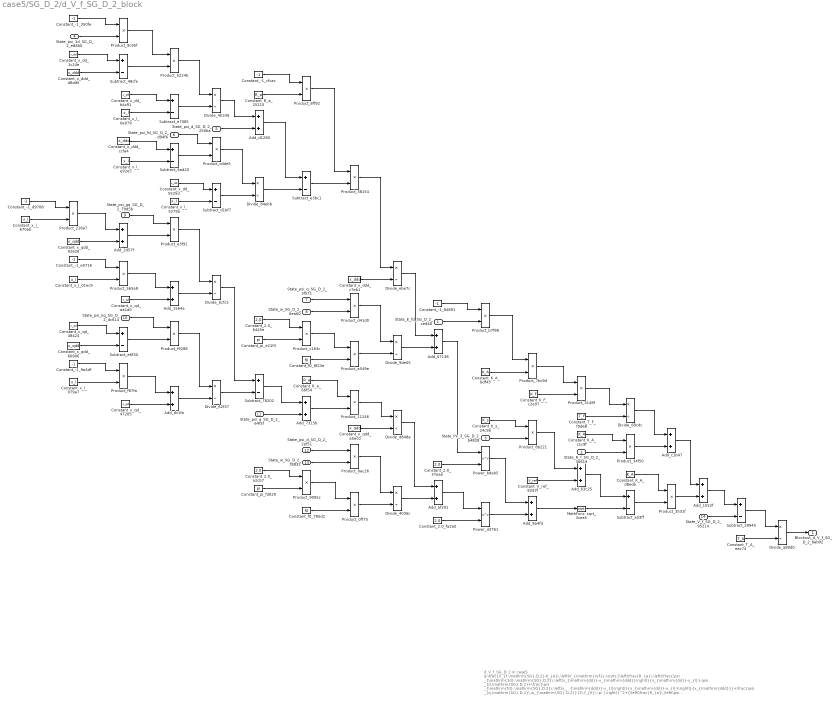
== system case5/SG_D_2/d_V_f_SG_D_2_block ==
  note: d_V_f_SG_D_2 in case5
      | $-\frac{V_{f,\mathrm{SG},D,2}-K_{A}\,\left(V_{\mathrm{ref}}-\sqrt{{\left(\frac{R_{a}\,\left(\frac{\psi _{\mathrm{1d},\mathrm{SG},D,2}\,\left(x_{\mathrm{dd}}-x_{\mathrm{ddd}}\right)}{x_{\mathrm{dd}}-x_{l}}-\psi _{d,\mathrm{SG},D,2}+\frac{\psi _{\mathrm{fd},\mathrm{SG},D,2}\,\left(x_{\mathrm{ddd}}-x_{l}\right)}{x_{\mathrm{dd}}-x_{l}}\right)}{x_{\mathrm{ddd}}}+\frac{\psi _{q,\mathrm{SG},D,2}\,w_{\mathrm{SG},D,2}}{2\,f_{0}\,\pi }\right)}^2+{\left(\frac{R_{a}\,\left(\psi _{q,\mathrm{SG},D,2}+\frac{\psi _{\mathrm{gq},\mathrm{SG},D,2}\,\left(x_{l}-x_{\mathrm{qdd}}\right)}{x_{l}-x_{\mathrm{qd}}}+\frac{\psi _{\mathrm{kq},\mathrm{SG},D,2}\,\left(x_{\mathrm{qd}}-x_{\mathrm{qdd}}\right)}{x_{l}-x_{\mathrm{qd}}}\right)}{x_{\mathrm{qdd}}}+\frac{\psi _{d,\mathrm{SG},D,2}\,w_{\mathrm{SG},D,2}}{2\,f_{0}\,\pi }\right)}^2}+K_{s}\,\mathrm{Px}_{3,\mathrm{SG},D,2}\right)-K_{A}\,R_{f,\mathrm{SG},D,2}+\frac{E_{\mathrm{fd},\mathrm{SG},D,2}\,K_{A}\,K_{F}}{T_{F}}}{T_{A}}$
      | Automatically generated on 2025-10-31 19:11:36 .
  State_E_fd_SG_D_2_ced48 : Inport
  State_R_f_SG_D_2_30619 : Inport  Port=2
  State_Px_3_SG_D_2_b4828 : Inport  Port=3
  State_psi_1d_SG_D_2_e8660 : Inport  Port=4
  State_psi_d_SG_D_2_250ba : Inport  Port=5
  State_psi_fd_SG_D_2_d94f6 : Inport  Port=6
  State_psi_q_SG_D_2_3f571 : Inport  Port=7
  State_w_SG_D_2_0ea60 : Inport  Port=8
  State_psi_gq_SG_D_2_79d5b : Inport  Port=9
  State_psi_kq_SG_D_2_dc614 : Inport  Port=10
  State_psi_q_SG_D_2_64f5f : Inport  Port=11
  State_psi_d_SG_D_2_2ef51 : Inport  Port=12
  State_w_SG_D_2_f8832 : Inport  Port=13
  State_V_f_SG_D_2_95214 : Inport  Port=14
  Add_1552f : Sum
  Add_1564a : Sum
  Add_2d57f : Sum
  Add_63c25 : Sum
  Add_67138 : Sum
  Add_7315b : Sum
  Add_8a4fd : Sum
  Add_af291 : Sum
  Add_c1b47 : Sum
  Add_d1280 : Sum
  Add_dc1fa : Sum
  Constant_-1_350fe : Constant  Value=-1
  Constant_-1_84891 : Constant  Value=-1
  Constant_-1_9a4df : Constant  Value=-1
  Constant_-1_cfcac : Constant  Value=-1
  Constant_-1_d9708 : Constant  Value=-1
  Constant_-1_e0716 : Constant  Value=-1
  Constant_2.0_37eae : Constant  Value=2.0
  Constant_2.0_6445e : Constant  Value=2.0
  Constant_2.0_a2cb7 : Constant  Value=2.0
  Constant_2.0_fa2a0 : Constant  Value=2.0
  Constant_K_A_bdf43 : Constant  Value=K_A
  Constant_K_A_c1c9f : Constant  Value=K_A
  Constant_K_A_d8ede : Constant  Value=K_A
  Constant_K_F_c2e97 : Constant  Value=K_F
  Constant_K_s_24c9b : Constant  Value=K_s
  Constant_R_a_25215 : Constant  Value=R_a
  Constant_R_a_66f54 : Constant  Value=R_a
  Constant_T_A_eac74 : Constant  Value=T_A
  Constant_T_F_f0d68 : Constant  Value=T_F
  Constant_V_ref_82d3f : Constant  Value=V_ref
  Constant_f0_785d2 : Constant  Value=f0
  Constant_f0_8f23e : Constant  Value=f0
  Constant_pi_e21f3 : Constant  Value=pi
  Constant_pi_fd029 : Constant  Value=pi
  Constant_x_dd_1c24e : Constant  Value=x_dd
  Constant_x_dd_5525d : Constant  Value=x_dd
  Constant_x_dd_b4c91 : Constant  Value=x_dd
  Constant_x_ddd_c7eb1 : Constant  Value=x_ddd
  Constant_x_ddd_ccfa4 : Constant  Value=x_ddd
  Constant_x_ddd_d8dd5 : Constant  Value=x_ddd
  Constant_x_l_01ec9 : Constant  Value=x_l
  Constant_x_l_079a7 : Constant  Value=x_l
  Constant_x_l_0e079 : Constant  Value=x_l
  Constant_x_l_5279a : Constant  Value=x_l
  Constant_x_l_670ab : Constant  Value=x_l
  Constant_x_l_e92e5 : Constant  Value=x_l
  Constant_x_qd_47205 : Constant  Value=x_qd
  Constant_x_qd_48424 : Constant  Value=x_qd
  Constant_x_qd_aa1a0 : Constant  Value=x_qd
  Constant_x_qdd_60906 : Constant  Value=x_qdd
  Constant_x_qdd_92628 : Constant  Value=x_qdd
  Constant_x_qdd_a5ec0 : Constant  Value=x_qdd
  Divide_4036c : Product  Inputs=*/
  Divide_4b336 : Product  Inputs=*/
  Divide_60cdc : Product  Inputs=*/
  Divide_62f37 : Product  Inputs=*/
  Divide_84ebb : Product  Inputs=*/
  Divide_9de05 : Product  Inputs=*/
  Divide_a80d0 : Product  Inputs=*/
  Divide_bcfc5 : Product  Inputs=*/
  Divide_d848a : Product  Inputs=*/
  Divide_ebe7c : Product  Inputs=*/
  MathFunc_sqrt_3cea5 : Sqrt
  Power_bdeb5 : Math  Operator=pow
  Power_d3761 : Math  Operator=pow
  Product_0ac26 : Product
  Product_0ff75 : Product
  Product_11246 : Product
  Product_218a7 : Product
  Product_3148f : Product
  Product_34f50 : Product
  Product_3531f : Product
  Product_38154 : Product
  Product_565a8 : Product
  Product_7bc9d : Product
  Product_8b221 : Product
  Product_8ff92 : Product
  Product_9095c : Product
  Product_9c9bf : Product
  Product_a549e : Product
  Product_b224b : Product
  Product_b7f88 : Product
  Product_c163c : Product
  Product_cdde5 : Product
  Product_d41d0 : Product
  Product_e3f91 : Product
  Product_f87fa : Product
  Product_f9288 : Product
  Subtract_29945 : Sum  Inputs=+-
  Subtract_48cfe : Sum  Inputs=+-
  Subtract_6ad20 : Sum  Inputs=+-
  Subtract_78202 : Sum  Inputs=+-
  Subtract_a03ff : Sum  Inputs=+-
  Subtract_d1bf7 : Sum  Inputs=+-
  Subtract_e3bc1 : Sum  Inputs=+-
  Subtract_e6f30 : Sum  Inputs=+-
  Subtract_e7085 : Sum  Inputs=+-
  Blockout_d_V_f_SG_D_2_8ab92 : Outport
  wires:
  Constant_-1_350fe/1 -> Product_9c9bf/1
  Constant_2.0_6445e/1 -> Product_c163c/1
  Constant_-1_d9708/1 -> Product_218a7/1
  Product_c163c/1 -> Product_a549e/1
  Product_218a7/1 -> Add_2d57f/1
  Constant_x_l_079a7/1 -> Product_f87fa/2
  Constant_x_l_670ab/1 -> Product_218a7/2
  State_psi_1d_SG_D_2_e8660/1 -> Product_9c9bf/2
  Constant_x_l_5279a/1 -> Subtract_d1bf7/2
  Constant_x_dd_1c24e/1 -> Subtract_48cfe/1
  Product_11246/1 -> Divide_d848a/1
  Constant_x_ddd_d8dd5/1 -> Subtract_48cfe/2
  Constant_x_qd_47205/1 -> Add_dc1fa/2
  Add_2d57f/1 -> Product_e3f91/2
  Constant_x_qdd_92628/1 -> Add_2d57f/2
  Constant_-1_e0716/1 -> Product_565a8/1
  Constant_x_dd_5525d/1 -> Subtract_d1bf7/1
  Subtract_78202/1 -> Add_7315b/1
  Power_bdeb5/1 -> Add_8a4fd/1
  Constant_x_l_01ec9/1 -> Product_565a8/2
  Constant_2.0_a2cb7/1 -> Product_9095c/1
  Constant_x_qd_48424/1 -> Subtract_e6f30/1
  Constant_pi_fd029/1 -> Product_9095c/2
  Subtract_e3bc1/1 -> Product_38154/2
  Constant_x_qdd_60906/1 -> Subtract_e6f30/2
  State_psi_fd_SG_D_2_d94f6/1 -> Product_cdde5/1
  Constant_-1_9a4df/1 -> Product_f87fa/1
  Product_9c9bf/1 -> Product_b224b/1
  State_w_SG_D_2_f8832/1 -> Product_0ac26/2
  Subtract_48cfe/1 -> Product_b224b/2
  Constant_x_dd_b4c91/1 -> Subtract_e7085/1
  State_psi_q_SG_D_2_64f5f/1 -> Add_7315b/2
  State_w_SG_D_2_0ea60/1 -> Product_d41d0/2
  Subtract_6ad20/1 -> Product_cdde5/2
  Constant_x_l_0e079/1 -> Subtract_e7085/2
  Add_c1b47/1 -> Add_1552f/1
  Constant_x_ddd_ccfa4/1 -> Subtract_6ad20/1
  Constant_x_l_e92e5/1 -> Subtract_6ad20/2
  State_psi_gq_SG_D_2_79d5b/1 -> Product_e3f91/1
  Product_565a8/1 -> Add_1564a/1
  Subtract_d1bf7/1 -> Divide_84ebb/2
  Constant_x_qd_aa1a0/1 -> Add_1564a/2
  Product_d41d0/1 -> Divide_9de05/1
  State_psi_kq_SG_D_2_dc614/1 -> Product_f9288/1
  Subtract_e6f30/1 -> Product_f9288/2
  Product_cdde5/1 -> Divide_84ebb/1
  State_V_f_SG_D_2_95214/1 -> Subtract_29945/2
  Product_f87fa/1 -> Add_dc1fa/1
  Product_b224b/1 -> Divide_4b336/1
  Divide_bcfc5/1 -> Subtract_78202/1
  Subtract_e7085/1 -> Divide_4b336/2
  Product_e3f91/1 -> Divide_bcfc5/1
  Add_1564a/1 -> Divide_bcfc5/2
  Product_f9288/1 -> Divide_62f37/1
  Divide_84ebb/1 -> Subtract_e3bc1/2
  Constant_f0_8f23e/1 -> Product_a549e/2
  Add_dc1fa/1 -> Divide_62f37/2
  Divide_4b336/1 -> Add_d1280/1
  State_psi_d_SG_D_2_250ba/1 -> Add_d1280/2
  Divide_62f37/1 -> Subtract_78202/2
  Constant_-1_cfcac/1 -> Product_8ff92/1
  Constant_R_a_25215/1 -> Product_8ff92/2
  Constant_f0_785d2/1 -> Product_0ff75/2
  Add_d1280/1 -> Subtract_e3bc1/1
  Product_8ff92/1 -> Product_38154/1
  Constant_pi_e21f3/1 -> Product_c163c/2
  State_psi_q_SG_D_2_3f571/1 -> Product_d41d0/1
  Constant_R_a_66f54/1 -> Product_11246/1
  State_E_fd_SG_D_2_ced48/1 -> Product_b7f88/2
  Add_7315b/1 -> Product_11246/2
  State_psi_d_SG_D_2_2ef51/1 -> Product_0ac26/1
  Product_9095c/1 -> Product_0ff75/1
  Product_38154/1 -> Divide_ebe7c/1
  Constant_x_ddd_c7eb1/1 -> Divide_ebe7c/2
  Product_a549e/1 -> Divide_9de05/2
  Constant_x_qdd_a5ec0/1 -> Divide_d848a/2
  Product_0ac26/1 -> Divide_4036c/1
  Product_0ff75/1 -> Divide_4036c/2
  Divide_ebe7c/1 -> Add_67138/1
  Divide_9de05/1 -> Add_67138/2
  Divide_d848a/1 -> Add_af291/1
  Divide_4036c/1 -> Add_af291/2
  Constant_-1_84891/1 -> Product_b7f88/1
  Add_67138/1 -> Power_bdeb5/1
  Constant_2.0_37eae/1 -> Power_bdeb5/2
  Add_af291/1 -> Power_d3761/1
  Constant_2.0_fa2a0/1 -> Power_d3761/2
  Product_b7f88/1 -> Product_7bc9d/1
  Constant_K_A_bdf43/1 -> Product_7bc9d/2
  Constant_K_s_24c9b/1 -> Product_8b221/1
  State_Px_3_SG_D_2_b4828/1 -> Product_8b221/2
  Power_d3761/1 -> Add_8a4fd/2
  Product_7bc9d/1 -> Product_3148f/1
  Constant_K_F_c2e97/1 -> Product_3148f/2
  Product_8b221/1 -> Add_63c25/1
  Constant_V_ref_82d3f/1 -> Add_63c25/2
  Add_8a4fd/1 -> MathFunc_sqrt_3cea5/1
  Product_3148f/1 -> Divide_60cdc/1
  Constant_T_F_f0d68/1 -> Divide_60cdc/2
  Constant_K_A_c1c9f/1 -> Product_34f50/1
  State_R_f_SG_D_2_30619/1 -> Product_34f50/2
  Add_63c25/1 -> Subtract_a03ff/1
  MathFunc_sqrt_3cea5/1 -> Subtract_a03ff/2
  Divide_60cdc/1 -> Add_c1b47/1
  Product_34f50/1 -> Add_c1b47/2
  Constant_K_A_d8ede/1 -> Product_3531f/1
  Subtract_a03ff/1 -> Product_3531f/2
  Product_3531f/1 -> Add_1552f/2
  Add_1552f/1 -> Subtract_29945/1
  Subtract_29945/1 -> Divide_a80d0/1
  Constant_T_A_eac74/1 -> Divide_a80d0/2
  Divide_a80d0/1 -> Blockout_d_V_f_SG_D_2_8ab92/1

== system case5/SG_D_2/d_psi_1d_SG_D_2_block ==
  note: d_psi_1d_SG_D_2 in case5
      | $-\frac{\psi _{\mathrm{1d},\mathrm{SG},D,2}-\psi _{\mathrm{fd},\mathrm{SG},D,2}+\frac{\left(x_{\mathrm{dd}}-x_{l}\right)\,\left(\frac{\psi _{\mathrm{1d},\mathrm{SG},D,2}\,\left(x_{\mathrm{dd}}-x_{\mathrm{ddd}}\right)}{x_{\mathrm{dd}}-x_{l}}-\psi _{d,\mathrm{SG},D,2}+\frac{\psi _{\mathrm{fd},\mathrm{SG},D,2}\,\left(x_{\mathrm{ddd}}-x_{l}\right)}{x_{\mathrm{dd}}-x_{l}}\right)}{x_{\mathrm{ddd}}}}{T_{\mathrm{ddd}}}$
      | Automatically generated on 2025-10-31 19:11:08 .
  State_psi_1d_SG_D_2_febab : Inport
  State_psi_fd_SG_D_2_ecfb2 : Inport  Port=2
  State_psi_1d_SG_D_2_31dd9 : Inport  Port=3
  State_psi_d_SG_D_2_bbb49 : Inport  Port=4
  State_psi_fd_SG_D_2_f55be : Inport  Port=5
  Add_4b4f4 : Sum
  Add_6ef35 : Sum
  Add_7724c : Sum
  Constant_-1_4bf4f : Constant  Value=-1
  Constant_-1_9b760 : Constant  Value=-1
  Constant_T_ddd_f1a03 : Constant  Value=T_ddd
  Constant_x_dd_08f8b : Constant  Value=x_dd
  Constant_x_dd_161a8 : Constant  Value=x_dd
  Constant_x_dd_5d104 : Constant  Value=x_dd
  Constant_x_dd_fa31b : Constant  Value=x_dd
  Constant_x_ddd_44fa1 : Constant  Value=x_ddd
  Constant_x_ddd_5b4ee : Constant  Value=x_ddd
  Constant_x_ddd_8ce00 : Constant  Value=x_ddd
  Constant_x_l_14552 : Constant  Value=x_l
  Constant_x_l_5048d : Constant  Value=x_l
  Constant_x_l_6eed4 : Constant  Value=x_l
  Constant_x_l_caf45 : Constant  Value=x_l
  Divide_699d9 : Product  Inputs=*/
  Divide_9b6a4 : Product  Inputs=*/
  Divide_9e3e9 : Product  Inputs=*/
  Divide_a3325 : Product  Inputs=*/
  Product_2c2d3 : Product
  Product_5b545 : Product
  Product_a4586 : Product
  Product_bcefe : Product
  Product_c02ff : Product
  Subtract_2b685 : Sum  Inputs=+-
  Subtract_454e5 : Sum  Inputs=+-
  Subtract_aced8 : Sum  Inputs=+-
  Subtract_b77a1 : Sum  Inputs=+-
  Subtract_cb346 : Sum  Inputs=+-
  Subtract_e4b08 : Sum  Inputs=+-
  Blockout_d_psi_1d_SG_D_2_44b96 : Outport
  wires:
  Subtract_2b685/1 -> Product_2c2d3/2
  Constant_x_l_caf45/1 -> Subtract_b77a1/2
  Divide_9e3e9/1 -> Add_7724c/2
  Subtract_cb346/1 -> Product_a4586/2
  Constant_-1_9b760/1 -> Product_5b545/1
  Constant_x_dd_5d104/1 -> Subtract_aced8/1
  Divide_a3325/1 -> Blockout_d_psi_1d_SG_D_2_44b96/1
  State_psi_fd_SG_D_2_ecfb2/1 -> Add_4b4f4/2
  State_psi_1d_SG_D_2_31dd9/1 -> Product_5b545/2
  Divide_699d9/1 -> Subtract_cb346/2
  Constant_x_ddd_44fa1/1 -> Subtract_aced8/2
  State_psi_1d_SG_D_2_febab/1 -> Product_c02ff/2
  Product_5b545/1 -> Product_bcefe/1
  Subtract_aced8/1 -> Product_bcefe/2
  Constant_x_dd_161a8/1 -> Subtract_b77a1/1
  Constant_x_ddd_8ce00/1 -> Subtract_2b685/1
  Constant_x_l_14552/1 -> Subtract_2b685/2
  Product_bcefe/1 -> Divide_9b6a4/1
  Subtract_b77a1/1 -> Divide_9b6a4/2
  State_psi_fd_SG_D_2_f55be/1 -> Product_2c2d3/1
  Constant_x_dd_08f8b/1 -> Subtract_454e5/1
  Constant_x_l_5048d/1 -> Subtract_e4b08/2
  Constant_x_l_6eed4/1 -> Subtract_454e5/2
  Constant_x_ddd_5b4ee/1 -> Divide_9e3e9/2
  Divide_9b6a4/1 -> Add_6ef35/1
  State_psi_d_SG_D_2_bbb49/1 -> Add_6ef35/2
  Product_2c2d3/1 -> Divide_699d9/1
  Subtract_454e5/1 -> Divide_699d9/2
  Constant_x_dd_fa31b/1 -> Subtract_e4b08/1
  Add_6ef35/1 -> Subtract_cb346/1
  Constant_-1_4bf4f/1 -> Product_c02ff/1
  Subtract_e4b08/1 -> Product_a4586/1
  Product_c02ff/1 -> Add_4b4f4/1
  Product_a4586/1 -> Divide_9e3e9/1
  Add_4b4f4/1 -> Add_7724c/1
  Add_7724c/1 -> Divide_a3325/1
  Constant_T_ddd_f1a03/1 -> Divide_a3325/2
